simulink model "bistable_and_rebound_plots"  (R2022a)
settings: Solver=VariableStepAuto  StartTime=0.0  StopTime=10.0  RelTol=1e-3
libraries: neuromorphic_blocks x5
settings Model: Creator=chris  LastModifiedBy=chris

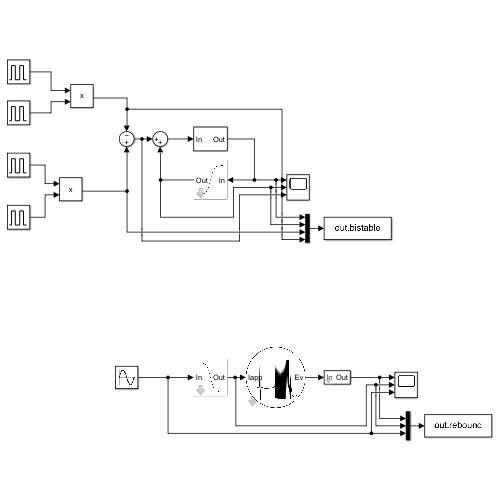
[thumbnail: Simulink's stored preview of the top-level diagram]
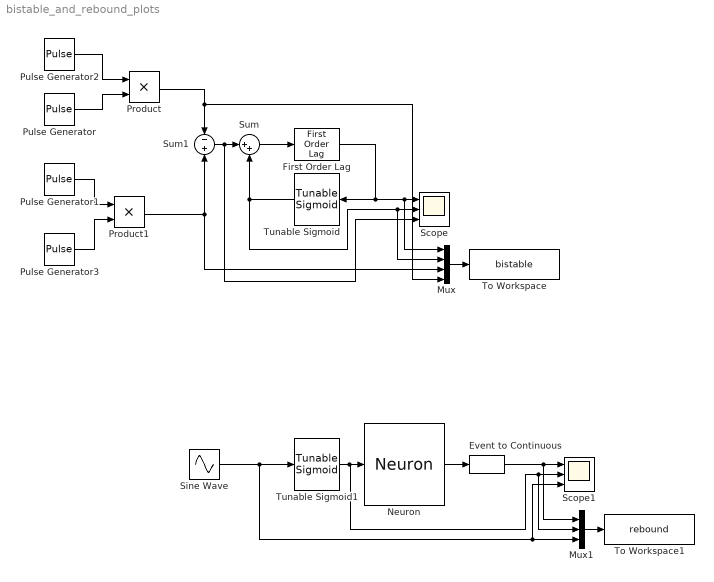
== system bistable_and_rebound_plots ==
  Event to Continuous : neuromorphic_blocks/Events Transmission Blocks/Event to Continuous  gain=1
      settings: SourceProductName=Neuromorphic Toolbox
  First Order Lag : neuromorphic_blocks/First Order Lag  gain=1  timescale=0.004  rel_timescale=1
      settings: SourceProductName=Neuromorphic Toolbox
  Mux : Mux
  Mux1 : Mux  Inputs=3
  Neuron : neuromorphic_blocks/Neural Blocks/Neuron  gfm_source=Internal  gfm=3  gsp_source=Internal  gsp=10  gsm_source=Internal  gsm=0  gup_source=Internal  gup=0  gum_source=Internal  gum=0  dfm=0  dsp=0.5  dsm=0  dup=0  dum=0  mfm=1  msp=1  msm=1  mup=1  mum=1  timescale=0.004  rel_membrane=0.1  rel_fast=0.1  rel_slow=4  rel_ultraslow=200  Iapp_base=0  V0=-1.2  tresh=0  output=Events
      settings: SourceProductName=Neuromorphic Toolbox
  Product : Product
  Product1 : Product
  Pulse Generator : DiscretePulseGenerator  PulseType=Time based  Amplitude=10  Period=0.5  PulseWidth=2  PhaseDelay=0.25
  Pulse Generator1 : DiscretePulseGenerator  PulseType=Time based  Amplitude=10  Period=0.5  PulseWidth=2
  Pulse Generator2 : DiscretePulseGenerator  PulseType=Time based  Period=5  PulseWidth=90  PhaseDelay=-2.5
  Pulse Generator3 : DiscretePulseGenerator  PulseType=Time based  Period=5  PulseWidth=75  PhaseDelay=2
  Scope : Scope  NumInputPorts=3
  Scope1 : Scope  NumInputPorts=3
  Sine Wave : Sin  Amplitude=5  Frequency=20  SampleTime=0
  Sum : Sum  Inputs=|++
  Sum1 : Sum  Inputs=-|+
  To Workspace : ToWorkspace  VariableName=bistable  SaveFormat=Structure With Time  SampleTime=0.001
  To Workspace1 : ToWorkspace  VariableName=rebound  SaveFormat=Structure With Time  SampleTime=0.001
  Tunable Sigmoid : neuromorphic_blocks/Tunable Sigmoid  nonlinearity_type=Tanh  gain_source=Internal  gain=5  bias=0  slope=1
      settings: SourceProductName=Neuromorphic Toolbox
  Tunable Sigmoid1 : neuromorphic_blocks/Tunable Sigmoid  nonlinearity_type=Sigmoid  gain_source=Internal  gain=-2  bias=0  slope=1
      settings: SourceProductName=Neuromorphic Toolbox
  wires:
  Sum/1 -> First Order Lag/1
  First Order Lag/1 -> Tunable Sigmoid/1, Mux/1, Scope/1
  Tunable Sigmoid/1 -> Mux/2, Scope/2, Sum/2
  Sum1/1 -> Scope/3, Sum/1
  Mux/1 -> To Workspace/1
  Tunable Sigmoid1/1 -> Mux1/2, Scope1/2, Neuron/1
  Sine Wave/1 -> Mux1/3, Scope1/3, Tunable Sigmoid1/1
  Neuron/1 -> Event to Continuous/1
  Mux1/1 -> To Workspace1/1
  Event to Continuous/1 -> Mux1/1, Scope1/1
  Pulse Generator/1 -> Product/2
  Pulse Generator2/1 -> Product/1
  Product/1 -> Mux/4, Sum1/1
  Pulse Generator1/1 -> Product1/1
  Pulse Generator3/1 -> Product1/2
  Product1/1 -> Mux/3, Sum1/2
